simulink model "cantoni_combined_matrices_3pools"  (R2019b)
settings: Solver=FixedStepDiscrete  StartTime=0.0  StopTime=1400  FixedStep=h  RelTol=1e-3
values from neighbouring files (symbols this model uses):
  comb_contr = ss(Ac, Bc, Cc, Dc, h)    [cantoni_LMI.m]
  comb_plant_disc = c2d(comb_plant_cont,h,'zoh')    [cantoni_LMI.m]
  h = 1    [cantoni_LMI.m]    (also in distributed_workspace.mat; model_hil.m = 0.00208333333333)
settings Model: Creator=Jacob  LastModifiedBy=bas
settings SFSimCC: CustomCodeUndefinedFunction=UseInterfaceOnly

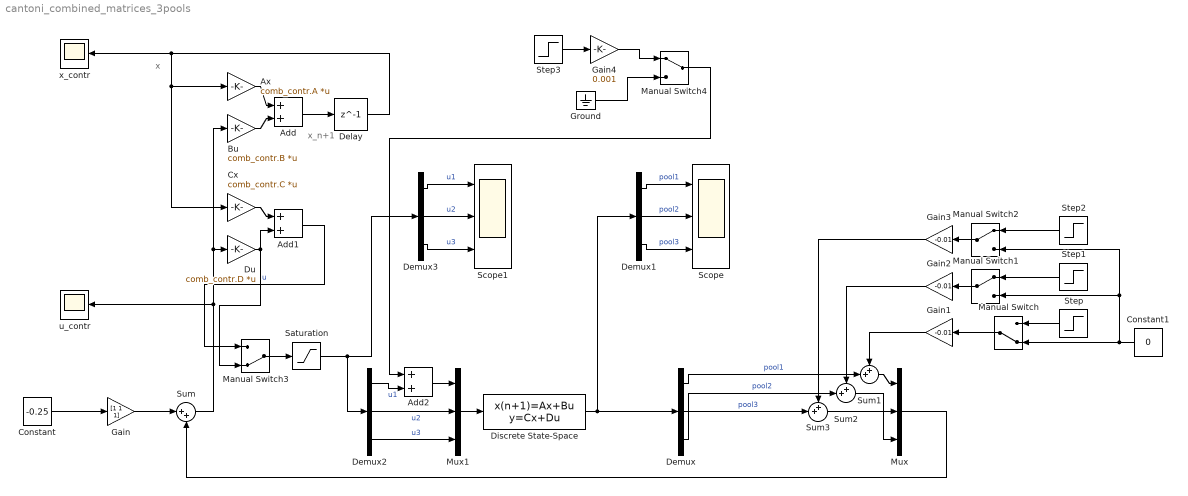
== system cantoni_combined_matrices_3pools ==
  note: x
  note: x_n+1
  Add : Sum
  Add1 : Sum
  Add2 : Sum
  Ax : Gain  Gain=comb_contr.A  Multiplication=Matrix(K*u)
  Bu : Gain  Gain=comb_contr.B  Multiplication=Matrix(K*u)
  Constant : Constant  Value=-0.25
  Constant1 : Constant  Value=0
  Cx : Gain  Gain=comb_contr.C  Multiplication=Matrix(K*u)
  Delay : Delay  DelayLength=1  InitialCondition=[0;0;0;0;0;0;0;0;0;0;0;0;0;0;0]
  Demux{,1..3} (4 alike) : Demux  Outputs=3
  Discrete State-Space : DiscreteStateSpace  A=comb_plant_disc.A  B=comb_plant_disc.B  C=comb_plant_disc.C  D=comb_plant_disc.D  SampleTime=h
  Du : Gain  Gain=comb_contr.D  Multiplication=Matrix(K*u)
  Gain : Gain  Gain=[1 1 1]
  Gain1 : Gain  Gain=-0.01
  Gain2 : Gain  Gain=-0.01
  Gain3 : Gain  Gain=-0.01
  Gain4 : Gain  Gain=0.001
  Ground : Ground
  Manual Switch : ManualSwitch  CurrentSetting=0
  Manual Switch1 : ManualSwitch
  Manual Switch2 : ManualSwitch
  Manual Switch3 : ManualSwitch  CurrentSetting=0
  Manual Switch4 : ManualSwitch
  Mux : Mux  Inputs=3
  Mux1 : Mux  Inputs=3
  Saturation : Saturate  UpperLimit=0.0035  LowerLimit=-0.0035
  Scope : Scope  NumInputPorts=3
  Scope1 : Scope  NumInputPorts=3
  Step : Step  Time=50  SampleTime=0
  Step1 : Step  Time=50  SampleTime=0
  Step2 : Step  Time=50  SampleTime=0
  Step3 : Step  SampleTime=0
  Sum : Sum  Inputs=|++
  Sum1 : Sum  Inputs=++|
  Sum2 : Sum  Inputs=++|
  Sum3 : Sum  Inputs=++|
  u_contr : Scope
  x_contr : Scope
  wires:
  Sum/1 -> Du/1, Bu/1, u_contr/1
  Discrete State-Space/1 -> Demux/1, Demux1/1
  Constant/1 -> Gain/1
  Gain/1 -> Sum/1
  Mux/1 -> Sum/2
  Demux1/1 -> Scope/1  "pool1"
  Demux1/2 -> Scope/2  "pool2"
  Demux1/3 -> Scope/3  "pool3"
  Step/1 -> Manual Switch/1
  Sum1/1 -> Mux/1
  Demux/2 -> Sum2/2  "pool2"
  Sum2/1 -> Mux/2
  Gain2/1 -> Sum2/1
  Step1/1 -> Manual Switch1/1
  Gain1/1 -> Sum1/1
  Manual Switch/1 -> Gain1/1
  Constant1/1 -> Manual Switch1/2, Manual Switch2/2, Manual Switch/2
  Manual Switch1/1 -> Gain2/1
  Demux/3 -> Sum3/2  "pool3"
  Sum3/1 -> Mux/3
  Manual Switch2/1 -> Gain3/1
  Step2/1 -> Manual Switch2/1
  Gain3/1 -> Sum3/1
  Demux/1 -> Sum1/2  "pool1"
  Mux1/1 -> Discrete State-Space/1
  Demux2/3 -> Mux1/3  "u3"
  Demux2/2 -> Mux1/2  "u2"
  Demux3/3 -> Scope1/3  "u3"
  Demux3/2 -> Scope1/2  "u2"
  Demux3/1 -> Scope1/1  "u1"
  Ax/1 -> Add/1
  Add/1 -> Delay/1
  Bu/1 -> Add/2
  Delay/1 -> x_contr/1, Cx/1, Ax/1
  Cx/1 -> Add1/1
  Du/1 -> Manual Switch3/2, Add1/2
  Add1/1 -> Manual Switch3/1  "u"
  Manual Switch3/1 -> Saturation/1
  Saturation/1 -> Demux2/1, Demux3/1
  Step3/1 -> Gain4/1
  Gain4/1 -> Manual Switch4/1
  Ground/1 -> Manual Switch4/2
  Demux2/1 -> Add2/2  "u1"
  Add2/1 -> Mux1/1
  Manual Switch4/1 -> Add2/1
